simulink model "TMS"  (R2023b)
settings: Solver=FixedStepDiscrete  StartTime=0.0  StopTime=10.0  FixedStep=0.1  RelTol=1e-3  EnableMultiTasking=on
settings Model: Creator=schro  LastModifiedBy=schro
settings SolverCC: AlgebraicLoopSolver=TrustRegion  AutoInsertRateTranBlk=on
settings DataIOCC: ExternalInput=[a.time, a.values]  LimitDataPoints=on  LoadExternalInput=on
settings OptimizationCC: LifeSpan=inf
settings DebuggingCC: UnconnectedInputMsg=warning  UnconnectedOutputMsg=warning  UnconnectedLineMsg=warning  AllowSymbolicDim=off  SFUnexpectedBacktrackingDiag=warning  SFNoUnconditionalDefaultTransitionDiag=warning  SFExecutionAtInitializationDiag=none  ArithmeticOperatorsInVariantConditions=warning
settings ModelReferenceCC: EnableRefExpFcnMdlSchedulingChecks=on
settings SFSimCC: SimUseLocalCustomCode=off  CustomCodeUndefinedFunction=UseInterfaceOnly
settings RTWCC: RTWUseLocalCustomCode=off  DLArmComputeVersion=19.05
settings CodeAppCC: StateflowObjectComments=on
settings GRTTargetCC: TargetLangStandard=C89/C90 (ANSI)
settings ConfigComp: CovMetricSettings=dw  CovSaveCumulativeToWorkspaceVar=on  CovSaveSingleToWorkspaceVar=on  CovExternalEMLEnable=off  CovSFcnEnable=off

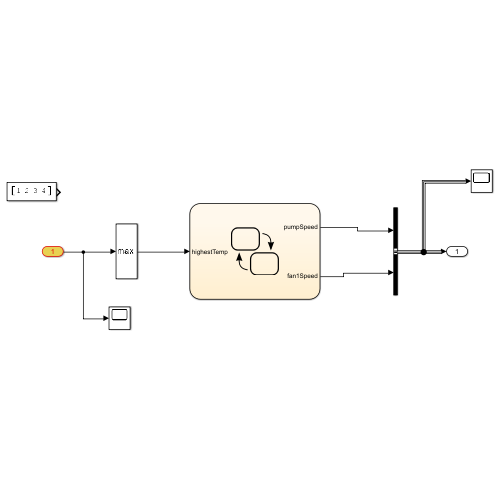
[thumbnail: Simulink's stored preview of the top-level diagram]
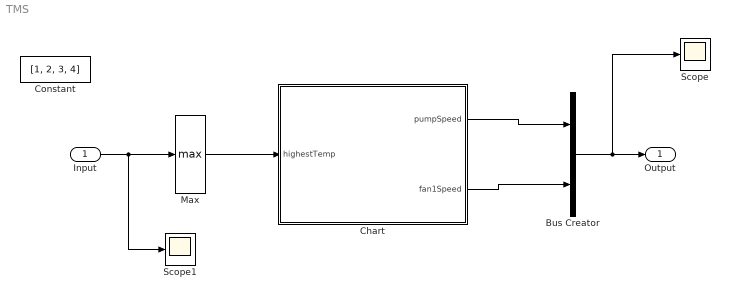
== system TMS ==
  Input : Inport
  Bus Creator : BusCreator  Inputs=2
  Chart : Stateflow chart  TreatAsAtomicUnit=on
  Constant : Constant  Value=[1, 2, 3, 4]  OutDataTypeStr=int8
  Max : MinMax  Function=max
  Scope : Scope
  Scope1 : Scope
  Output : Outport
  wires:
  Chart/1(pumpSpeed) -> Bus Creator/1
  Chart/2(fan1Speed) -> Bus Creator/2
  Bus Creator/1 -> Scope/1, Output/1
  Max/1 -> Chart/1(highestTemp)
  Input/1 -> Scope1/1, Max/1

== stateflow chart TMS/Chart ==
  state COOL_LEVEL_MAX
    pumpSpeed = 100;
    fan1Speed = 100;
  state COOL_LEVEL_1
    pumpSpeed = 75;
    fan1Speed = 75;
  state COOL_LEVEL_2
    pumpSpeed = 50;
    fan1Speed = 50;
  state COOL_LEVEL_IDLE
    pumpSpeed = 50;
    fan1Speed = 0;
  COOL_LEVEL_MAX -> COOL_LEVEL_IDLE
  COOL_LEVEL_1 -> COOL_LEVEL_MAX [order 1] : [highestTemp >= 50]
  COOL_LEVEL_1 -> COOL_LEVEL_IDLE [order 2] : [highestTemp < 50]
  COOL_LEVEL_2 -> COOL_LEVEL_1 [order 1] : [highestTemp >=40]
  COOL_LEVEL_2 -> COOL_LEVEL_IDLE [order 2] : [highestTemp < 40]
  COOL_LEVEL_IDLE -> COOL_LEVEL_2 : [highestTemp >= 30]
  (default) -> COOL_LEVEL_IDLE
  data: pumpSpeed output; fan1Speed output; highestTemp input
